simulink model "AEB_KPI_Project"  (R2025a)
settings: Solver=VariableStepAuto  StartTime=0.0  StopTime=10.0  RelTol=1e-3
settings Model: Creator=wangjianhai  LastModifiedBy=wangjianhai

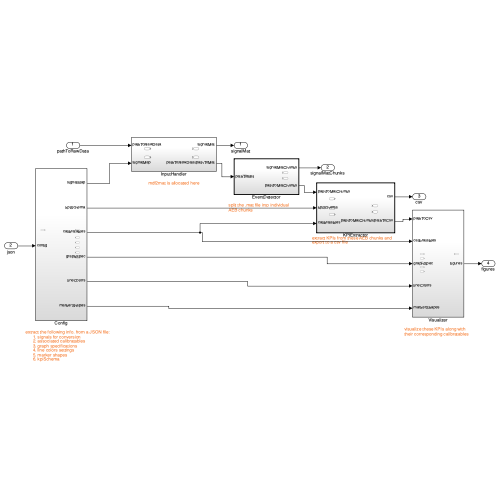
[thumbnail: Simulink's stored preview of the top-level diagram]
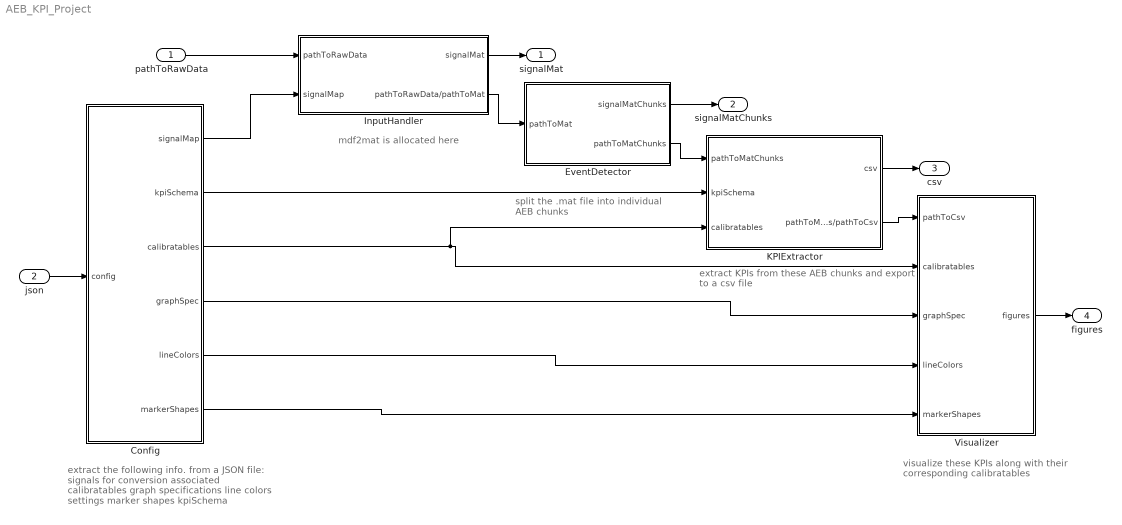
== system AEB_KPI_Project ==
  note: extract the following info. from a JSON file:
      | signals for conversion
      | associated calibratables
      | graph specifications
      | line colors settings
      | marker shapes
      | kpiSchema
  note: visualize these KPIs along with their corresponding calibratables
  note: extract KPIs from these AEB chunks and export to a csv file
  note: split the .mat file into individual AEB chunks
  note: mdf2mat is allocated here
  pathToRawData : Inport
  json : Inport  Port=2
  Config : Subsystem
  EventDetector : Subsystem  TreatAsAtomicUnit=on
  InputHandler : Subsystem
  KPIExtractor : Subsystem  AutoFrameSizeCalculation=on
  Visualizer : Subsystem
  signalMat : Outport  VectorParamsAs1DForOutWhenUnconnected=off
  signalMatChunks : Outport  Port=2  VectorParamsAs1DForOutWhenUnconnected=off
  csv : Outport  Port=3  VectorParamsAs1DForOutWhenUnconnected=off
  figures : Outport  Port=4  VectorParamsAs1DForOutWhenUnconnected=off
  wires:
  Visualizer/1(figures) -> figures/1
  Config/6(markerShapes) -> Visualizer/5(markerShapes)
  Config/5(lineColors) -> Visualizer/4(lineColors)
  Config/4(graphSpec) -> Visualizer/3(graphSpec)
  InputHandler/2(pathToRawData/pathToMat) -> EventDetector/1(pathToMat)
  KPIExtractor/1(csv) -> csv/1
  Config/2(kpiSchema) -> KPIExtractor/2(kpiSchema)
  EventDetector/1(signalMatChunks) -> signalMatChunks/1
  InputHandler/1(signalMat) -> signalMat/1
  EventDetector/2(pathToMatChunks) -> KPIExtractor/1(pathToMatChunks)
  Config/1(signalMap) -> InputHandler/2(signalMap)
  pathToRawData/1 -> InputHandler/1(pathToRawData)
  KPIExtractor/2(pathToMatChunks/pathToCsv) -> Visualizer/1(pathToCsv)
  Config/3(calibratables) -> KPIExtractor/3(calibratables), Visualizer/2(calibratables)
  json/1 -> Config/1(config)

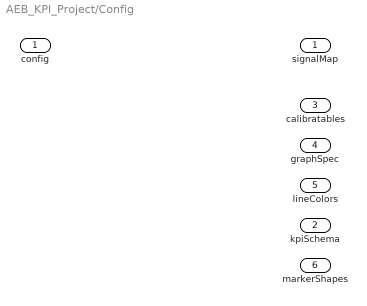
== system AEB_KPI_Project/Config ==
  config : Inport
  signalMap : Outport
  kpiSchema : Outport  Port=2
  calibratables : Outport  Port=3
  graphSpec : Outport  Port=4
  lineColors : Outport  Port=5
  markerShapes : Outport  Port=6

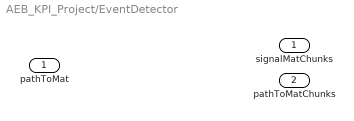
== system AEB_KPI_Project/EventDetector ==
  pathToMat : Inport
  signalMatChunks : Outport
  pathToMatChunks : Outport  Port=2

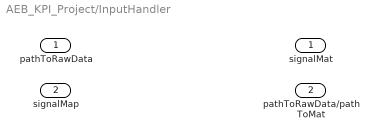
== system AEB_KPI_Project/InputHandler ==
  pathToRawData : Inport
  signalMap : Inport  Port=2
  signalMat : Outport
  pathToRawData/pathToMat : Outport  Port=2

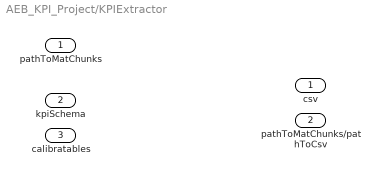
== system AEB_KPI_Project/KPIExtractor ==
  pathToMatChunks : Inport
  kpiSchema : Inport  Port=2
  calibratables : Inport  Port=3
  csv : Outport  VectorParamsAs1DForOutWhenUnconnected=off
  pathToMatChunks/pathToCsv : Outport  Port=2  VectorParamsAs1DForOutWhenUnconnected=off

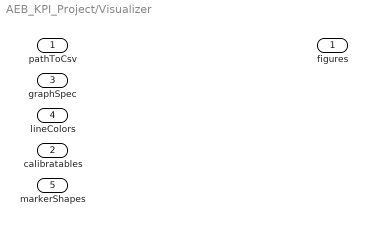
== system AEB_KPI_Project/Visualizer ==
  pathToCsv : Inport
  calibratables : Inport  Port=2
  graphSpec : Inport  Port=3
  lineColors : Inport  Port=4
  markerShapes : Inport  Port=5
  figures : Outport
